simulink model "two_link_model_invdynamic"  (R2021a)
settings: Solver=ode45  StartTime=0.0  StopTime=20  RelTol=1e-3  EnableMultiTasking=on
model workspace (MAT data in the model file):
  q_d_start = [0 0]
  q_d_stop = [1.57079632679 1.57079632679]
undefined symbols (not defined in the file or in its folder): F, f, K_D, K_P
settings Model: OrderedModelArguments=off  Creator=kma  LastModifiedBy=frida
settings SolverCC: AlgebraicLoopSolver=TrustRegion
settings DataIOCC: LimitDataPoints=on  SaveFormat=Array  ReturnWorkspaceOutputs=off
settings OptimizationCC: LifeSpan=inf
settings DebuggingCC: SFUnexpectedBacktrackingDiag=warning  SFNoUnconditionalDefaultTransitionDiag=warning  SFExecutionAtInitializationDiag=none  SFMachineParentedDataDiag=warning  ArithmeticOperatorsInVariantConditions=warning
settings HardwareCC: ProdBitPerPointer=32  ProdBitPerSizeT=32  ProdBitPerPtrDiffT=32  ProdLargestAtomicFloat=None  ProdIntDivRoundTo=Undefined  ProdEndianess=Unspecified  ProdWordSize=32  ProdHWDeviceType=32-bit Generic
settings ModelReferenceCC: PropagateSignalLabelsOutOfModel=off
settings SFSimCC: SimUseLocalCustomCode=off  CustomCodeUndefinedFunction=UseInterfaceOnly
settings RTWCC: RTWUseLocalCustomCode=off
settings CodeAppCC: StateflowObjectComments=on
settings GRTTargetCC: TargetLangStandard=C89/C90 (ANSI)
settings ConfigComp: CovMetricSettings=dw  CovSaveCumulativeToWorkspaceVar=on  CovSaveSingleToWorkspaceVar=on  CovExternalEMLEnable=off

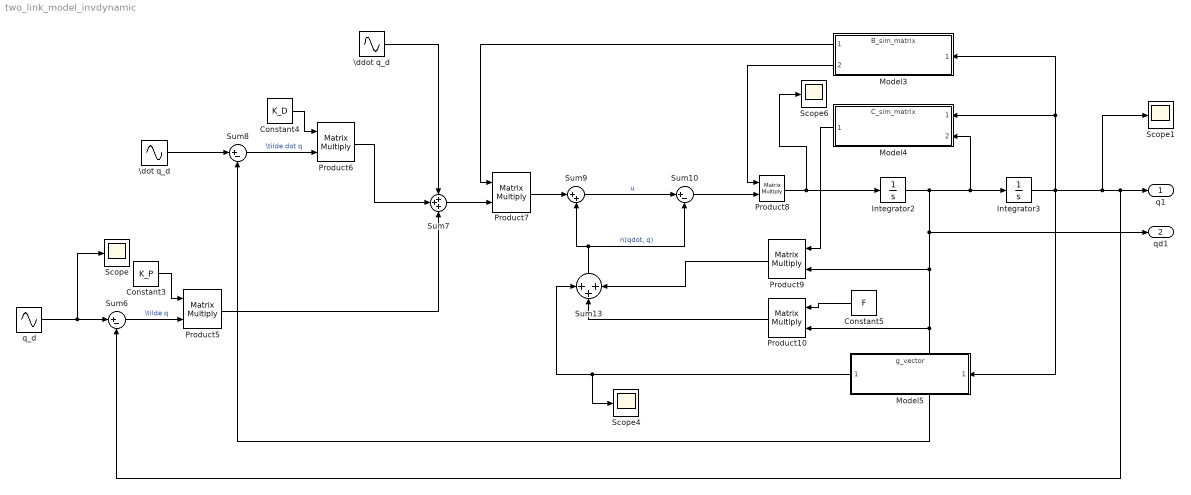
== system two_link_model_invdynamic ==
  Constant3 : Constant  Value=K_P
  Constant4 : Constant  Value=K_D
  Constant5 : Constant  Value=F
  Integrator2 : Integrator
  Integrator3 : Integrator
  Model3 : ModelReference  ModelNameDialog=B_sim_matrix.slx  SimulationMode=Normal  ModelReferenceVersion=1.6
  Model4 : ModelReference  ModelNameDialog=C_sim_matrix.slx  SimulationMode=Normal  ModelReferenceVersion=1.2
  Model5 : ModelReference  ModelNameDialog=g_vector.slx  SimulationMode=Normal  ModelReferenceVersion=1.8
  Product{5..10} (6 alike) : Product  Multiplication=Matrix(*)
  Scope{,1,4,6} (4 alike) : Scope
  Sum10 : Sum  Inputs=|+-
  Sum13 : Sum  Inputs=+++
  Sum6 : Sum  Inputs=|+-
  Sum7 : Sum  Inputs=+++
  Sum8 : Sum  Inputs=|+-
  Sum9 : Sum  Inputs=|++
  \ddot q_d : Sin  Amplitude=-4*(pi^2)*(f^2)  Frequency=[2*pi*f, 2*pi*f]  SampleTime=0
  \dot q_d : Sin  Amplitude=2*pi*f  Frequency=[2*pi*f, 2*pi*f]  Phase=pi/2  SampleTime=0
  q_d : Sin  Frequency=[2*pi*f, 2*pi*f]  SampleTime=0
  q1 : Outport  PortDimensions=2
  qd1 : Outport  Port=2  PortDimensions=2
  wires:
  Constant4/1 -> Product6/1
  Sum8/1 -> Product6/2  "\\tilde dot q"
  Product7/1 -> Sum9/1
  Product5/1 -> Sum7/3
  Sum6/1 -> Product5/2  "\\tilde q"
  Product6/1 -> Sum7/2
  \ddot q_d/1 -> Sum7/1
  Sum7/1 -> Product7/2
  Constant3/1 -> Product5/1
  Model5/1 -> Scope4/1, Sum13/1
  Product10/1 -> Sum13/2
  Product8/1 -> Scope6/1, Integrator2/1
  Constant5/1 -> Product10/1
  Integrator2/1 -> Sum8/2, Product10/2, Product9/2, qd1/1, Model4/2, Integrator3/1
  Product9/1 -> Sum13/3
  Integrator3/1 -> Sum6/2, q1/1, Scope1/1, Model5/1, Model3/1, Model4/1
  Model4/1 -> Product9/1
  Model3/2 -> Product8/1
  Model3/1 -> Product7/1
  Sum13/1 -> Sum9/2, Sum10/2  "n(qdot, q)"
  Sum9/1 -> Sum10/1  "u"
  Sum10/1 -> Product8/2
  \dot q_d/1 -> Sum8/1
  q_d/1 -> Scope/1, Sum6/1
